simulink model "Continuous_System_1"  (R2023a)
settings: Solver=VariableStepAuto  StartTime=0.0  StopTime=10.0  RelTol=1e-3
undefined symbols (not defined in the file): r
settings Model: Creator=Aman  LastModifiedBy=Aman

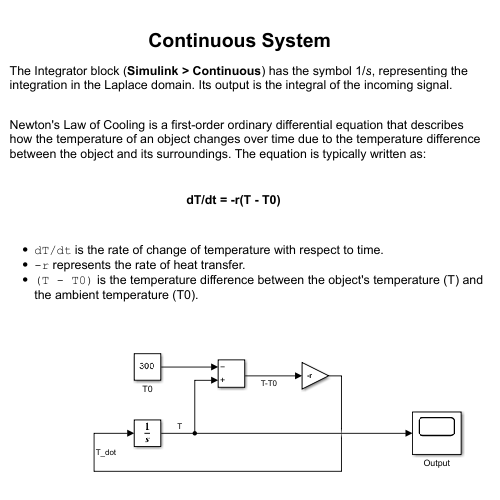
[thumbnail: Simulink's stored preview of the top-level diagram]
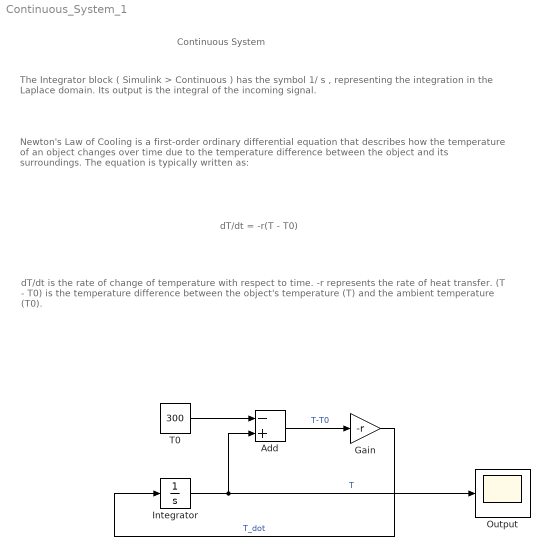
== system Continuous_System_1 ==
  note: dT/dt is the rate of change of temperature with respect to time.
      | -r represents the rate of heat transfer.
      | (T - T0) is the temperature difference between the object's temperature (T) and the ambient temperature (T0).
  note: dT/dt = -r(T - T0)
  note: Newton's Law of Cooling is a first-order ordinary differential equation that describes how the temperature of an object changes over time due to the temperature difference between the object and its surroundings. The equation is typically written as:
  note: The Integrator block ( Simulink > Continuous ) has the symbol 1/ s , representing the integration in the Laplace domain. Its output is the integral of the incoming signal.
  note: Continuous System
  Add : Sum  Inputs=-+
  Gain : Gain  Gain=-r
  Integrator : Integrator  InitialCondition=320
  Output : Scope
  T0 : Constant  Value=300
  wires:
  Gain/1 -> Integrator/1  "T_dot"
  Add/1 -> Gain/1  "T-T0"
  Integrator/1 -> Output/1, Add/2  "T"
  T0/1 -> Add/1
